simulink model "normalpid"  (R2018b)
settings: Solver=VariableStepAuto  StartTime=0.0  StopTime=50.0  RelTol=1e-3
values from neighbouring files (symbols this model uses):
  xcos = 0:10    [variables.m]
  ycos = 0:10    [variables.m]
libraries: simulink x2
settings Model: Creator=axelwillekens  LastModifiedBy=axelwillekens

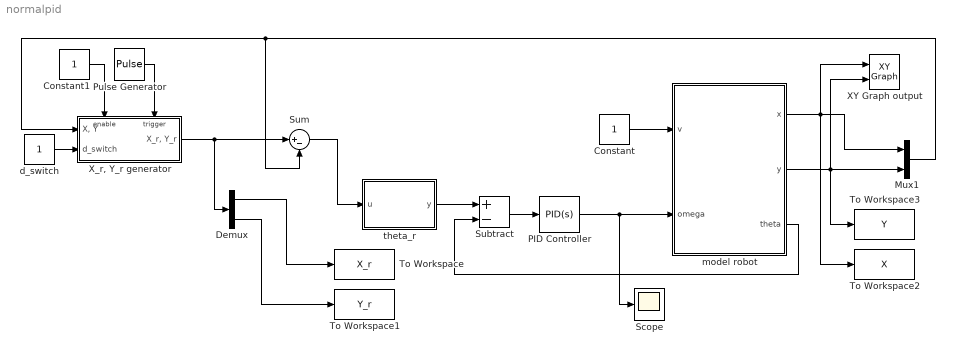
== system normalpid ==
  Constant : Constant
  Constant1 : Constant
  Demux : Demux  Outputs=2
  Mux1 : Mux  Inputs=2
  PID Controller : simulink/Continuous/PID Controller  Controller=PID  Form=Parallel  TimeDomain=Continuous-time  SampleTime=-1  IntegratorMethod=Forward Euler  FilterMethod=Forward Euler  ControllerParametersSource=internal  P=3  I=0.9  D=3  UseFilter=on  N=100  TunerSelectOption=Transfer Function Based (PID Tuner App)  InitialConditionSource=internal  InitialConditionForIntegrator=0  InitialConditionForFilter=0  DifferentiatorICPrevScaledInput=0  ExternalReset=none  TrackingMode=off  Kt=1  LimitOutput=off  UpperSaturationLimit=pi/4  LowerSaturationLimit=-pi/4  LinearizeAsGain=on  AntiWindupMode=none  Kb=1  POutMin=[]  POutMax=[]  IOutMin=[]  IOutMax=[]  DOutMin=[]  DOutMax=[]  NOutMin=[]  NOutMax=[]  SumOutMin=[]  SumOutMax=[]  SaturationOutMin=[]  SaturationOutMax=[]  PParamMin=[]  PParamMax=[]  IParamMin=[]  IParamMax=[]  DParamMin=[]  DParamMax=[]  NParamMin=[]  NParamMax=[]  KbParamMin=[]  KbParamMax=[]  KtParamMin=[]  KtParamMax=[]  KbOutMin=[]  KbOutMax=[]  KtOutMin=[]  KtOutMax=[]  IntegratorOutMin=[]  IntegratorOutMax=[]  FilterOutMin=[]  FilterOutMax=[]  SumI1OutMin=[]  SumI1OutMax=[]  SumI2OutMin=[]  SumI2OutMax=[]  SumI3OutMin=[]  SumI3OutMax=[]  SumI4OutMin=[]  SumI4OutMax=[]  SumDOutMin=[]  SumDOutMax=[]  DifferentiatorOutMin=[]  DifferentiatorOutMax=[]  FilterDiffOutCoefMin=[]  FilterDiffOutCoefMax=[]  ReciprocalOutMin=[]  ReciprocalOutMax=[]  SumDenOutMin=[]  SumDenOutMax=[]  SumNumOutMin=[]  SumNumOutMax=[]  DivideOutMin=[]  DivideOutMax=[]  IntegratorContinuousStateAttributes=''  IntegratorStateMustResolveToSignalObject=off  IntegratorRTWStateStorageClass=Auto  FilterContinuousStateAttributes=''  FilterStateMustResolveToSignalObject=off  FilterRTWStateStorageClass=Auto  ParallelPVariant=InternalParameters  IdealPVariant=Disabled  IVariant=InternalParameters  DVariant=InternalParameters  IntegratorVariant=Continuous  SatVariant=Disabled  AWVariant=Passthrough  PCopyVariant=Disabled  TRVariant=Disabled  FdbkBlocksVariant=Forward  IdealPFdbkVariant=Disabled  SatFdbkVariant=Disabled  DerivativeFilterVariant=ContFilter  NVariant=InternalParameters  NCopyVariant=Disabled  FilterICVariant=InternalICsFilter  IntegratorICVariant=InternalICs  ExternalResetVariant=Disabled  TRSumVariant=Passthrough  SumFdbkVariant=Disabled  SumVariant=Sum_PID
  Pulse Generator : DiscretePulseGenerator  PulseType=Time based  Period=0.05  PulseWidth=5
  Scope : Scope
  Subtract : Sum  Inputs=+-
  Sum : Sum  Inputs=|+-
  To Workspace : ToWorkspace  VariableName=X_r  SaveFormat=Timeseries  SampleTime=-1
  To Workspace1 : ToWorkspace  VariableName=Y_r  SaveFormat=Timeseries  SampleTime=-1
  To Workspace2 : ToWorkspace  VariableName=X  SaveFormat=Timeseries  SampleTime=-1
  To Workspace3 : ToWorkspace  VariableName=Y  SaveFormat=Timeseries  SampleTime=-1
  XY Graph output : simulink/Sinks/XY Graph  xmin=-2  xmax=15  ymin=-2  ymax=15  st=-1
  "X_r, Y_r generator" : Subsystem  TreatAsAtomicUnit=on
  d_switch : Constant
  model robot : Subsystem
  theta_r : MATLAB Function  TreatAsAtomicUnit=on
  wires:
  d_switch/1 -> "X_r, Y_r generator"/2(d_switch)
  model robot/2(y) -> XY Graph output/2, To Workspace3/1, Mux1/2
  Demux/2 -> To Workspace1/1
  Pulse Generator/1 -> "X_r, Y_r generator"/Trigger
  Constant1/1 -> "X_r, Y_r generator"/Enable
  "X_r, Y_r generator"/1("X_r, Y_r") -> Demux/1, Sum/1
  model robot/3(theta) -> Subtract/2
  Demux/1 -> To Workspace/1
  PID Controller/1 -> Scope/1, model robot/2(omega)
  Subtract/1 -> PID Controller/1
  Sum/1 -> theta_r/1(u)
  Mux1/1 -> "X_r, Y_r generator"/1("X, Y"), Sum/2
  theta_r/1(y) -> Subtract/1
  model robot/1(x) -> XY Graph output/1, To Workspace2/1, Mux1/1
  Constant/1 -> model robot/1(v)

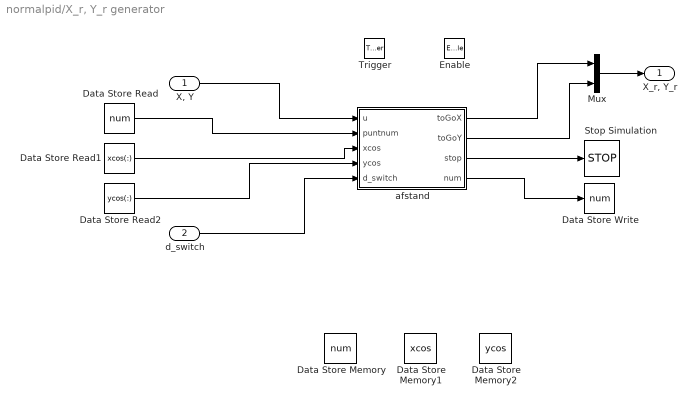
== system normalpid/X_r, Y_r generator ==
  "X, Y" : Inport
  d_switch : Inport  Port=2
  Enable : EnablePort
  Trigger : TriggerPort  VariantControl=Variant
  Data Store Memory : DataStoreMemory  DataStoreName=num  ReadBeforeWriteMsg=warning  WriteAfterWriteMsg=warning  WriteAfterReadMsg=warning  InitialValue=1  ShowAdditionalParam=off
  Data Store Memory1 : DataStoreMemory  DataStoreName=xcos  ReadBeforeWriteMsg=warning  WriteAfterWriteMsg=warning  WriteAfterReadMsg=warning  InitialValue=linspace(0,100,101)  ShowAdditionalParam=off
  Data Store Memory2 : DataStoreMemory  DataStoreName=ycos  ReadBeforeWriteMsg=warning  WriteAfterWriteMsg=warning  WriteAfterReadMsg=warning  InitialValue=linspace(0,100,101)  ShowAdditionalParam=off
  Data Store Read : DataStoreRead  DataStoreName=num  DataStoreElements=num
  Data Store Read1 : DataStoreRead  DataStoreName=xcos  DataStoreElements=xcos(:)
  Data Store Read2 : DataStoreRead  DataStoreName=ycos  DataStoreElements=ycos(:)
  Data Store Write : DataStoreWrite  DataStoreName=num  DataStoreElements=num
  Mux : Mux  Inputs=2
  Stop Simulation : Stop
  afstand : MATLAB Function  TreatAsAtomicUnit=on
  "X_r, Y_r" : Outport
  wires:
  "X, Y"/1 -> afstand/1(u)
  afstand/1(toGoX) -> Mux/1
  afstand/3(stop) -> Stop Simulation/1
  Data Store Read/1 -> afstand/2(puntnum)
  afstand/4(num) -> Data Store Write/1
  Data Store Read1/1 -> afstand/3(xcos)
  Data Store Read2/1 -> afstand/4(ycos)
  afstand/2(toGoY) -> Mux/2
  Mux/1 -> "X_r, Y_r"/1
  d_switch/1 -> afstand/5(d_switch)

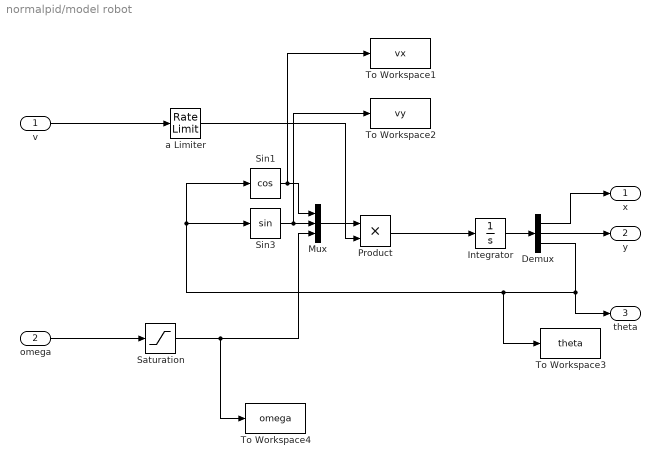
== system normalpid/model robot ==
  v : Inport
  omega : Inport  Port=2
  Demux : Demux  Outputs=3
  Integrator : Integrator  InitialCondition=[0 0 -pi/4]
  Mux : Mux  Inputs=3
  Product : Product
  Saturation : Saturate  UpperLimit=50*(pi/180)  LowerLimit=-50*(pi/180)
  Sin1 : Trigonometry  Operator=cos
  Sin3 : Trigonometry
  To Workspace1 : ToWorkspace  VariableName=vx  SaveFormat=Timeseries  SampleTime=-1
  To Workspace2 : ToWorkspace  VariableName=vy  SaveFormat=Timeseries  SampleTime=-1
  To Workspace3 : ToWorkspace  VariableName=theta  SaveFormat=Timeseries  SampleTime=-1
  To Workspace4 : ToWorkspace  VariableName=omega  SaveFormat=Timeseries  SampleTime=-1
  a Limiter : RateLimiter  SampleTimeMode=inherited
  x : Outport
  y : Outport  Port=2
  theta : Outport  Port=3
  wires:
  a Limiter/1 -> Product/2
  Mux/1 -> Product/1
  Product/1 -> Integrator/1
  Integrator/1 -> Demux/1
  Demux/2 -> y/1
  Demux/1 -> x/1
  Demux/3 -> To Workspace3/1, Sin3/1, Sin1/1, theta/1
  Sin1/1 -> To Workspace1/1, Mux/1
  omega/1 -> Saturation/1
  Sin3/1 -> Mux/2, To Workspace2/1
  v/1 -> a Limiter/1
  Saturation/1 -> To Workspace4/1, Mux/3

== matlab function normalpid/theta_r ==
  data: u input; y output
function y = fcn(u)

y = atan2(u(2),u(1));

== matlab function normalpid/X_r, Y_r generator/afstand ==
  data: u input; toGoX output; toGoY output; stop output; puntnum input; num output; xcos input; ycos input; d_switch input
function [toGoX, toGoY, stop, num] = fcn(u, puntnum, xcos, ycos, d_switch)
d = sqrt((xcos(puntnum)-u(1))^2 + (ycos(puntnum)-u(2))^2);
if d < d_switch
    num = puntnum + 1;
else
    num = puntnum;
end

toGoX = xcos(puntnum); 
toGoY = ycos(puntnum);

if num > length(xcos)
    stop = 1;
else
    stop = 0;
end
